simulink library "INP_KEY_EB"  (R2023b)
settings: Solver=VariableStepAuto  StartTime=0.0  StopTime=10.0  RelTol=1e-3
settings Model: Creator=blatak  LastModifiedBy=blatak

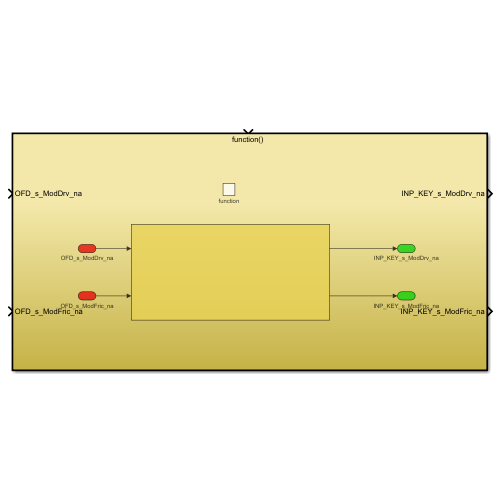
[thumbnail: Simulink's stored preview of the top-level diagram]
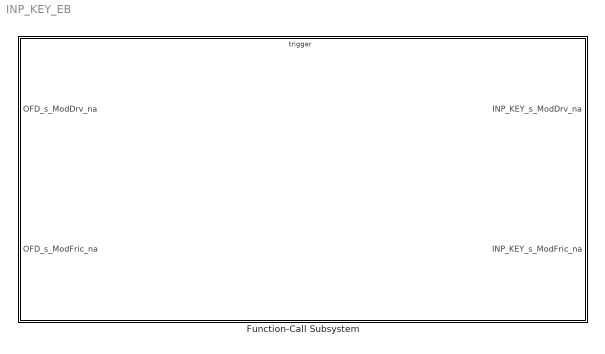
== system INP_KEY_EB ==
  Function-Call Subsystem : Subsystem  TreatAsAtomicUnit=on

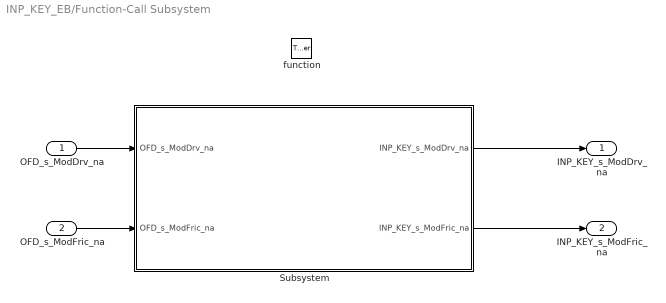
== system INP_KEY_EB/Function-Call Subsystem ==
  OFD_s_ModDrv_na : Inport
  OFD_s_ModFric_na : Inport  Port=2
  function : TriggerPort  TriggerType=function-call  VariantControl=(inherit)
  Subsystem : Subsystem
  INP_KEY_s_ModDrv_na : Outport
  INP_KEY_s_ModFric_na : Outport  Port=2
  wires:
  OFD_s_ModDrv_na/1 -> Subsystem/1(OFD_s_ModDrv_na)
  OFD_s_ModFric_na/1 -> Subsystem/2(OFD_s_ModFric_na)
  Subsystem/1(INP_KEY_s_ModDrv_na) -> INP_KEY_s_ModDrv_na/1
  Subsystem/2(INP_KEY_s_ModFric_na) -> INP_KEY_s_ModFric_na/1

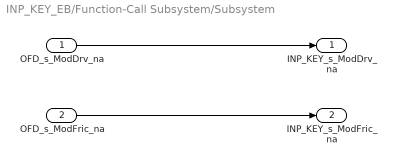
== system INP_KEY_EB/Function-Call Subsystem/Subsystem ==
  OFD_s_ModDrv_na : Inport
  OFD_s_ModFric_na : Inport  Port=2
  INP_KEY_s_ModDrv_na : Outport
  INP_KEY_s_ModFric_na : Outport  Port=2
  wires:
  OFD_s_ModDrv_na/1 -> INP_KEY_s_ModDrv_na/1
  OFD_s_ModFric_na/1 -> INP_KEY_s_ModFric_na/1
